simulink model "blockdemo"  (Simulink 6.3)
settings: Solver=FixedStepDiscrete  StartTime=0.0  StopTime=20.0  RelTol=1e-3
InitFcn:
  | %% DSPBuilder Start
  | alt_dspbuilder_update_model(bdroot)
  | %% DSPBuilder End
libraries: allblocks_alteradspbuilder2 x7
settings Model: Creator=cpurcell  LastModifiedBy=delphick
settings DebuggingCC: MultiTaskDSMMsg=error

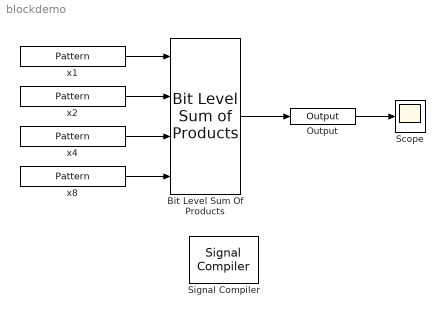
== system blockdemo ==
  Bit Level Sum Of Products : allblocks_alteradspbuilder2/Bit Level Sum of Products  number_of_coefficients=4  BusType=Signed Integer  bwl=8  bwr=0  coefficients=[1 2 4 8]  register_inputs=on  use_ena=off  use_sclr=off
  Output : allblocks_alteradspbuilder2/Output  iofile=C:\workspace_clean\Documentation\DesignExamples\Tutorials\UnitBlocks\Arithmetic\BitLevelSumOfProducts\tb_blockdemo\blockdemo_Output.capture  BusType=Signed Integer  bwl=10  bwr=0  PORTTYPE=Output
  Scope : Scope
      settings: TimeRange=20  YMin=-1  YMax=16
  Signal Compiler : allblocks_alteradspbuilder2/Signal Compiler  DeviceFamily=Stratix IV  DeviceName=AUTO  EnableSignalTap=off  SignalTapDepth=128  UseBoardBlock=off  StpUseDefaultClock=on  StpClock=clock
  x1 : allblocks_alteradspbuilder2/Pattern  Sequence=0101010101010101  SpecifyClock=off  use_ena=off  use_sclr=off
  x2 : allblocks_alteradspbuilder2/Pattern  Sequence=0011001100110011  SpecifyClock=off  use_ena=off  use_sclr=off
  x4 : allblocks_alteradspbuilder2/Pattern  Sequence=0000111100001111  SpecifyClock=off  use_ena=off  use_sclr=off
  x8 : allblocks_alteradspbuilder2/Pattern  Sequence=0000000011111111  SpecifyClock=off  use_ena=off  use_sclr=off
  wires:
  x1/1 -> Bit Level Sum Of Products/1
  x2/1 -> Bit Level Sum Of Products/2
  x4/1 -> Bit Level Sum Of Products/3
  x8/1 -> Bit Level Sum Of Products/4
  Bit Level Sum Of Products/1 -> Output/1
  Output/1 -> Scope/1
